simulink model "mpc_doubleint"  (Simulink 5.0)
settings: Solver=ode45  SolverMode=SingleTasking  StartTime=0.0  StopTime=5  RelTol=1e-3
values from neighbouring files (symbols this model uses):
  r = ones(Tf,1)    [misosim.m]    (also in misoss.m = 1; mpcoffsets.m = r0*ones(Tf,1))
undefined symbols (not defined in the file or in its folder): x01, x02
libraries: mpclib x1
settings Model: LastModifiedBy=Alberto Bemporad  ExtModeTrigMode=oneshot  ExtModeArmWhenConnect=off  LimitDataPoints=off  IntegerOverflowMsg=none  BooleanDataType=off  ZeroCrossControl=UseLocalSettings  RTWMathFcnLibMatFile=iso_c_tmw.mat  RTWOptions="-aEnforceIntegerDowncast=1 -aFoldNonRolledExpr=1 -aInlineInvariantSignals=1 -aInlineParameters=0 -aLocalBlockOutputs=1 -aRollThreshold=5 -aRTWVerbose=1 -aForceParamTrailComments=0 -aGenerateComments=1 -aIgnoreCustomStorageClasses=1 -aIncHierarchyInIds=0 -aMaxRTWIdLen=31 -aShowEliminatedStatements=0 -aReadOnly=0 -aTargetFcnLib=\"iso_c_tmw.mat\" -aIncDataTypeInIds=0 -aPrefixModelToSubsysFcnNames=1 -aInlinedPrmAccess=\"Literals\" -aGenerateFullHeader=1 -aIsPILTarget=0 -aGenerateReport=0 -aLogVarNameModifier=\"rt_\" -aExtMode=0 -aExtModeStaticAlloc=0 -aExtModeTesting=0 -aExtModeStaticAllocSize=1000000 -aExtModeTransport=0"

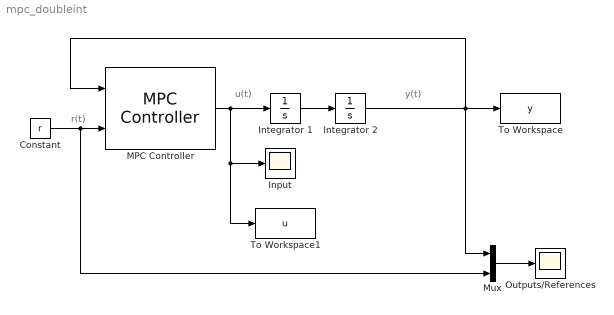
== system mpc_doubleint ==
  note: u(t)
  note: y(t)
  note: r(t)
  Constant : Constant  Value=r
  Input : Scope
      settings: TimeRange=6  YMin=-1  YMax=1  DataFormat=Structure
  Integrator 1 : Integrator  InitialCondition=x01  UpperSaturationLimit=Inf  LowerSaturationLimit=-Inf
  Integrator 2 : Integrator  InitialCondition=x02  UpperSaturationLimit=Inf  LowerSaturationLimit=-Inf
  MPC Controller : mpclib/MPC Controller  mpcobj=mpc_controller  x0=[]  ref_from_ws=off  ref_signal_name=[]  ref_preview=on  md_from_ws=off  md_signal_name=[]  md_preview=on
      link override Mux: Inputs=2
  Mux : Mux  Inputs=2
  Outputs/References : Scope
      settings: TimeRange=5  YMin=0  YMax=1.5  DataFormat=Structure
  To Workspace : ToWorkspace  VariableName=y  SampleTime=-1  SaveFormat=Array
      settings: MaxDataPoints=Inf
  To Workspace1 : ToWorkspace  VariableName=u  SampleTime=-1  SaveFormat=Array
      settings: MaxDataPoints=Inf
  wires:
  MPC Controller/1 -> Integrator 1/1, Input/1, To Workspace1/1
  Integrator 2/1 -> To Workspace/1, Mux/1, MPC Controller/1
  Mux/1 -> Outputs/References/1
  Constant/1 -> Mux/2, MPC Controller/2
  Integrator 1/1 -> Integrator 2/1
